simulink model "FAst_MPC"  (R2016b)
settings: Solver=FixedStepAuto  StartTime=0.0  StopTime=30  FixedStep=Ts  RelTol=1e-3
values from neighbouring files (symbols this model uses):
  A = A_d    [Fast_MPC.m]
  B = B_d    [Fast_MPC.m]
  C = C_d    [Fast_MPC.m]
  D = D_d    [Fast_MPC.m]
  G1 = G1+K(:,i:i+1)*C*V(i)    [Fast_MPC.m]
  G2 = G2+K(:,i:i+1)*C*A^i    [Fast_MPC.m]
  Ke = Ke+K(:,i:i+1)    [Fast_MPC.m]
  Ts = 0.02    [Fast_MPC.m]
libraries: simulink x2
settings Model: Creator=Ashraf  LastModifiedBy=Ashraf

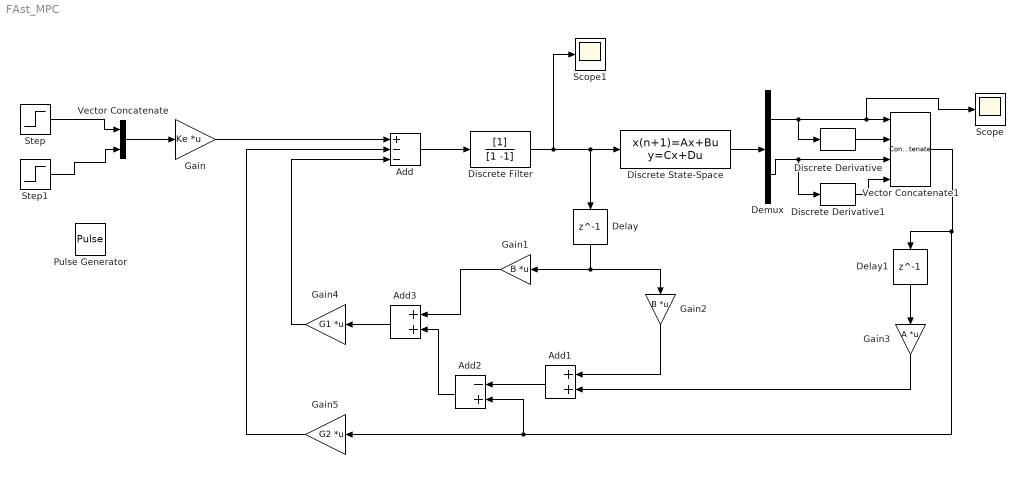
== system FAst_MPC ==
  Add : Sum  Inputs=+--
  Add1 : Sum
  Add2 : Sum  Inputs=-+
  Add3 : Sum
  Delay : Delay  DelayLength=1  SampleTime=Ts
  Delay1 : Delay  DelayLength=1  SampleTime=Ts
  Demux : Demux  Outputs=2
  Discrete Derivative : simulink/Discrete/Discrete Derivative  gainval=1.0  ICPrevScaledInput=0.0  OutMin=[]  OutMax=[]  OutDataType=fixdt(1, 16)  OutScaling=2^-10  DoSatur=off
  Discrete Derivative1 : simulink/Discrete/Discrete Derivative  gainval=1.0  ICPrevScaledInput=0.0  OutMin=[]  OutMax=[]  OutDataType=fixdt(1, 16)  OutScaling=2^-10  DoSatur=off
  Discrete Filter : DiscreteFilter  Denominator=[1 -1]  SampleTime=Ts
  Discrete State-Space : DiscreteStateSpace  A=A  B=B  C=C  D=D  SampleTime=Ts
  Gain : Gain  Gain=Ke  Multiplication=Matrix(K*u)
  Gain1 : Gain  Gain=B  Multiplication=Matrix(K*u)
  Gain2 : Gain  Gain=B  Multiplication=Matrix(K*u)
  Gain3 : Gain  Gain=A  Multiplication=Matrix(K*u)
  Gain4 : Gain  Gain=G1  Multiplication=Matrix(K*u)
  Gain5 : Gain  Gain=G2  Multiplication=Matrix(K*u)
  Pulse Generator : DiscretePulseGenerator  PulseType=Time based  Period=10  PulseWidth=5
  Scope : Scope
  Scope1 : Scope
  Step : Step  After=0.1  SampleTime=Ts
  Step1 : Step  After=0.1  SampleTime=Ts
  Vector Concatenate : Concatenate
  Vector Concatenate1 : Concatenate  NumInputs=4
  wires:
  Discrete Filter/1 -> Scope1/1, Discrete State-Space/1, Delay/1
  Step/1 -> Vector Concatenate/1
  Step1/1 -> Vector Concatenate/2
  Vector Concatenate/1 -> Gain/1
  Gain/1 -> Add/1
  Add/1 -> Discrete Filter/1
  Delay/1 -> Gain2/1, Gain1/1
  Discrete State-Space/1 -> Demux/1
  Delay1/1 -> Gain3/1
  Gain2/1 -> Add1/1
  Gain3/1 -> Add1/2
  Add1/1 -> Add2/1
  Gain1/1 -> Add3/1
  Add2/1 -> Add3/2
  Add3/1 -> Gain4/1
  Gain4/1 -> Add/3
  Gain5/1 -> Add/2
  Demux/2 -> Discrete Derivative1/1, Vector Concatenate1/3
  Demux/1 -> Discrete Derivative/1, Scope/1, Vector Concatenate1/1
  Discrete Derivative/1 -> Vector Concatenate1/2
  Discrete Derivative1/1 -> Vector Concatenate1/4
  Vector Concatenate1/1 -> Add2/2, Gain5/1, Delay1/1
